simulink model "parallel2ser2par"  (R2013b)
settings: Solver=VariableStepDiscrete  StartTime=0.0  StopTime=1e-3  FixedStep=simulationTime  RelTol=1e-3
undefined symbols (not defined in the file or in its folder): periSam, sampleTime
libraries: simulink x3, dspswit3 x1, powerlib_meascontrol x1
settings Model: Creator=mainster  LastModifiedBy=mainster

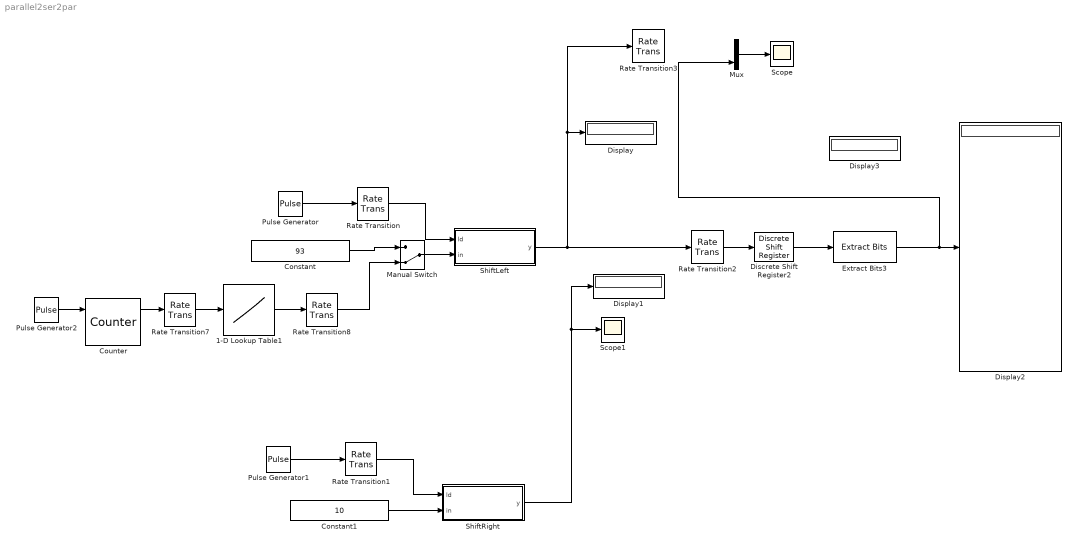
== system parallel2ser2par ==
  " ShiftLeft" : Subsystem  TreatAsAtomicUnit=on
  " ShiftRight" : Subsystem  TreatAsAtomicUnit=on
  1-D Lookup Table1 : Lookup_n-D  NumberOfTableDimensions=1  BreakpointsForDimension1=[0,1,2,3,4]  IndexSearchMethod=Evenly spaced points  UseOneInputPortForAllInputData=on  Table=[3325,6553,44558,8856,60254]  TableDataTypeStr=uint16  InterpMethod=Flat  SampleTime=sampleTime  InternalRulePriority=Speed  OutDataTypeStr=uint16  RndMeth=Simplest  InputSameDT=on
  Constant : Constant  Value=93  VectorParams1D=off  SampleTime=-1
  Constant1 : Constant  Value=10  VectorParams1D=off  SampleTime=-1
      settings: SamplingMode=Frame based
  Counter : dspswit3/Counter  Direction=Up  CountEvent=Rising edge  CounterSize=User defined  MaxCount=5  InitialCount=1  Output=Count and Hit  HitValue=32  ResetInput=on  SamplesPerFrame=1  Ts=1  CntDtype=double  HitDtype=Logical
  Discrete Shift Register2 : powerlib_meascontrol/Additional Components/Discrete Shift Register  NSamples=15  InitialValue=0  Ts=-1
  Display{,1..3} (4 alike) : Display
      settings: Format=binary (Stored Integer)
  Extract Bits3 : simulink/Logic and Bit Operations/Extract Bits  bitsToExtract=Range of bits  numBits=8  bitIdxRange=[0 0]  outScalingMode=Treat bit field as an integer
  Manual Switch : ManualSwitch  CurrentSetting=0
  Mux : Mux  Inputs=2
  Pulse Generator : DiscretePulseGenerator
  Pulse Generator1 : DiscretePulseGenerator
  Pulse Generator2 : DiscretePulseGenerator  Period=periSam*16  PulseWidth=8*periSam  SampleTime=sampleTime
  Rate Transition : RateTransition  OutPortSampleTime=0.1
  Rate Transition1 : RateTransition  OutPortSampleTime=0.1
  Rate Transition2 : RateTransition  OutPortSampleTime=1
  Rate Transition3 : RateTransition  OutPortSampleTime=1
  Rate Transition7 : RateTransition  OutPortSampleTime=sampleTime
  Rate Transition8 : RateTransition  OutPortSampleTime=sampleTime
  Scope : Scope
      settings: ShowLegends=on  TimeRange=0.001  YMin=94762.03896404211  YMax=95462.26442363281
  Scope1 : Scope
      settings: ShowLegends=on  TimeRange=0.001
  wires:
  " ShiftLeft"/1(y) -> Rate Transition2/1, Rate Transition3/1, Display/1
  Pulse Generator/1 -> Rate Transition/1
  Rate Transition/1 -> " ShiftLeft"/1(ld)
  Constant1/1 -> " ShiftRight"/2(in)
  " ShiftRight"/1(y) -> Display1/1, Scope1/1
  Pulse Generator1/1 -> Rate Transition1/1
  Rate Transition1/1 -> " ShiftRight"/1(ld)
  Discrete Shift Register2/1 -> Extract Bits3/1
  Rate Transition2/1 -> Discrete Shift Register2/1
  Extract Bits3/1 -> Mux/2, Display2/1
  Mux/1 -> Scope/1
  Rate Transition7/1 -> 1-D Lookup Table1/1
  1-D Lookup Table1/1 -> Rate Transition8/1
  Pulse Generator2/1 -> Counter/1
  Counter/1 -> Rate Transition7/1
  Constant/1 -> Manual Switch/1
  Rate Transition8/1 -> Manual Switch/2
  Manual Switch/1 -> " ShiftLeft"/2(in)

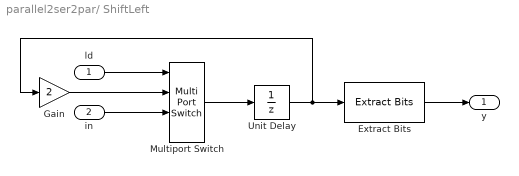
== system parallel2ser2par/ ShiftLeft ==
  ld : Inport
  in : Inport  Port=2
  Extract Bits : simulink/Logic and Bit Operations/Extract Bits  bitsToExtract=Range of bits  numBits=8  bitIdxRange=[15 15]  outScalingMode=Treat bit field as an integer
  Gain : Gain  Gain=2  ParamDataTypeStr=Inherit: Inherit from 'Gain'
  Multiport Switch : MultiPortSwitch  DataPortOrder=Zero-based contiguous  DiagnosticForDefault=Warning
  Unit Delay : UnitDelay  SampleTime=-1
  y : Outport
  wires:
  ld/1 -> Multiport Switch/1
  in/1 -> Multiport Switch/3
  Gain/1 -> Multiport Switch/2
  Multiport Switch/1 -> Unit Delay/1
  Unit Delay/1 -> Gain/1, Extract Bits/1
  Extract Bits/1 -> y/1

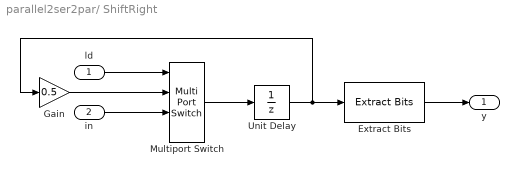
== system parallel2ser2par/ ShiftRight ==
  ld : Inport
  in : Inport  Port=2
  Extract Bits : simulink/Logic and Bit Operations/Extract Bits  bitsToExtract=Range of bits  numBits=8  bitIdxRange=[0 0]  outScalingMode=Treat bit field as an integer
  Gain : Gain  Gain=0.5  ParamDataTypeStr=Inherit: Inherit from 'Gain'
  Multiport Switch : MultiPortSwitch  DataPortOrder=Zero-based contiguous  DiagnosticForDefault=Warning
  Unit Delay : UnitDelay  SampleTime=-1
  y : Outport
  wires:
  ld/1 -> Multiport Switch/1
  in/1 -> Multiport Switch/3
  Gain/1 -> Multiport Switch/2
  Multiport Switch/1 -> Unit Delay/1
  Unit Delay/1 -> Gain/1, Extract Bits/1
  Extract Bits/1 -> y/1
